simulink model "Modele_Non_Lineaire_Asservi"  (R2024a)
settings: Solver=FixedStepAuto  StartTime=0.0  StopTime=30  FixedStep=0.01  RelTol=1e-3
values from neighbouring files (symbols this model uses):
  delay = 0    [Code.m]
  den_mot_simu = [R_m*J_eq  (R_m*B_eq+n_g*n_m*k_m*k_t*K_g.^2)]    [Code.m]    (also in Initialisation.m)
  Fig_in = 1    [Code.m]
  Frequence = pi    (= 3.14159265359)    [Code.m]
  g = 9.81    [Code.m]    (also in Initialisation.m)
  K_int = real((((-1)*den_mot(1)*(Inter^2)) + ((-1)*den_mot(2)*(Inter^1))) / (num_mot(1)))    [Code.m]    (also in Initialisation.m)
  L_plaque = 0.2750/2    (= 0.1375)    [Code.m]    (also in Initialisation.m = 0.275)
  num_mot_simu = [K_g*n_m*n_g*k_t]    [Code.m]    (also in Initialisation.m)
  r_arm = 0.0254    [Code.m]    (also in Initialisation.m)
  step_size = 0.01    [Code.m]
  Test_Position = 0.06    [Code.m]    (also in Initialisation.m)
  X_den = TF_PD_Bode_Den    [Code.m]    (also in Initialisation.m)
  X_num = TF_PD_Bode_Num    [Code.m]    (also in Initialisation.m)
settings Model: Creator=Mathys  LastModifiedBy=francoisdesautels
settings RTWCC: GPUComputeCapability=3.5

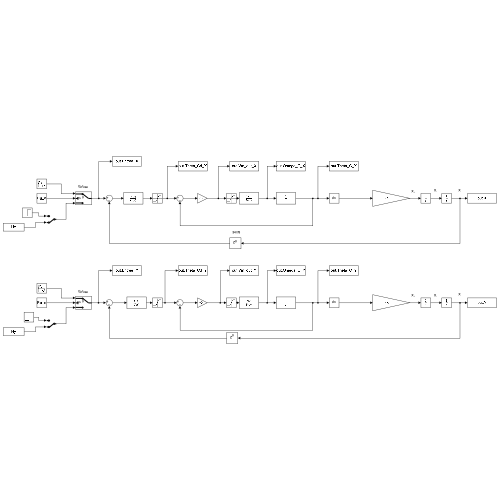
[thumbnail: Simulink's stored preview of the top-level diagram]
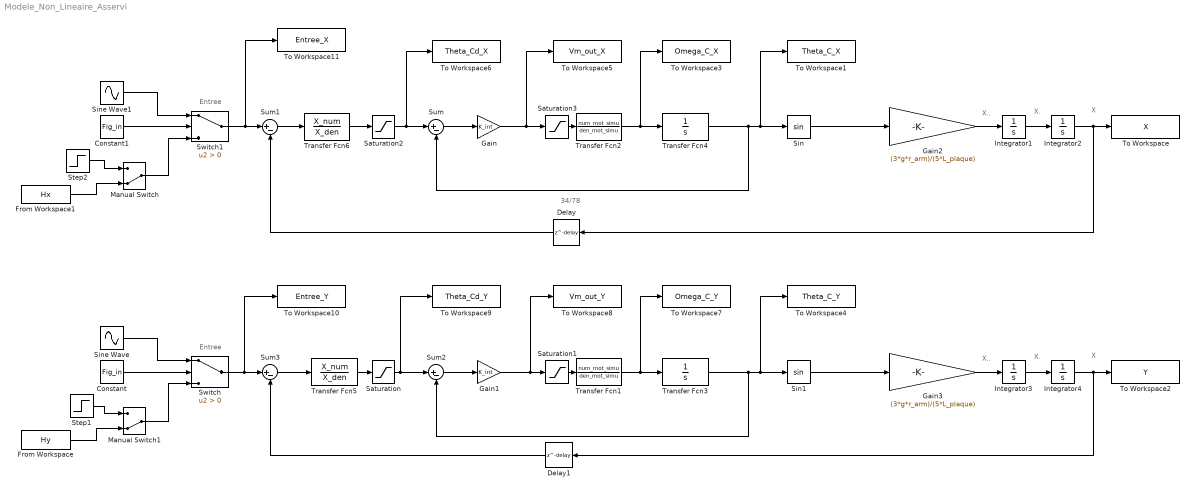
== system Modele_Non_Lineaire_Asservi ==
  note: 34/78
  note: X
  note: X.
  note: X..
  note: X..
  note: X.
  note: Entree
  note: X
  note: Entree
  Constant : Constant  Value=Fig_in
  Constant1 : Constant  Value=Fig_in
  Delay : Delay  DelayLength=delay
  Delay1 : Delay  DelayLength=delay
  From Workspace : FromWorkspace  VariableName=Hy  SampleTime=step_size
  From Workspace1 : FromWorkspace  VariableName=Hx  SampleTime=step_size
  Gain : Gain  Gain=K_int
  Gain1 : Gain  Gain=K_int
  Gain2 : Gain  Gain=(3*g*r_arm)/(5*L_plaque)
  Gain3 : Gain  Gain=(3*g*r_arm)/(5*L_plaque)
  Integrator{1..4} (4 alike) : Integrator
  Manual Switch : ManualSwitch  CurrentSetting=0
  Manual Switch1 : ManualSwitch  CurrentSetting=0
  Saturation : Saturate  UpperLimit=deg2rad(35)  LowerLimit=deg2rad(-35)
  Saturation1 : Saturate  UpperLimit=7.5  LowerLimit=-7.5
  Saturation2 : Saturate  UpperLimit=deg2rad(35)  LowerLimit=deg2rad(-35)
  Saturation3 : Saturate  UpperLimit=7.5  LowerLimit=-7.5
  Sin : Trigonometry
  Sin1 : Trigonometry
  Sine Wave : Sin  Amplitude=Test_Position  Frequency=Frequence  SampleTime=0
  Sine Wave1 : Sin  Amplitude=Test_Position  Frequency=Frequence  SampleTime=0
  Step1 : Step  After=Test_Position  SampleTime=0
  Step2 : Step  After=Test_Position  SampleTime=0
  Sum{,1..3} (4 alike) : Sum  Inputs=|+-
  Switch : Switch  Criteria=u2 > Threshold  SaturateOnIntegerOverflow=off  InputSameDT=off
  Switch1 : Switch  Criteria=u2 > Threshold  SaturateOnIntegerOverflow=off  InputSameDT=off
  To Workspace : ToWorkspace  VariableName=X  SampleTime=-1
  To Workspace1 : ToWorkspace  VariableName=Theta_C_X  SaveFormat=Timeseries  SampleTime=-1
      settings: Save2DSignal=2-D array (concatenate along first dimension)
  To Workspace10 : ToWorkspace  VariableName=Entree_Y  SaveFormat=Timeseries  SampleTime=-1
      settings: Save2DSignal=2-D array (concatenate along first dimension)
  To Workspace11 : ToWorkspace  VariableName=Entree_X  SaveFormat=Timeseries  SampleTime=-1
      settings: Save2DSignal=2-D array (concatenate along first dimension)
  To Workspace2 : ToWorkspace  VariableName=Y  SampleTime=-1
  To Workspace3 : ToWorkspace  VariableName=Omega_C_X  SampleTime=-1
  To Workspace4 : ToWorkspace  VariableName=Theta_C_Y  SaveFormat=Timeseries  SampleTime=-1
      settings: Save2DSignal=2-D array (concatenate along first dimension)
  To Workspace5 : ToWorkspace  VariableName=Vm_out_X  SaveFormat=Timeseries  SampleTime=-1
      settings: Save2DSignal=2-D array (concatenate along first dimension)
  To Workspace6 : ToWorkspace  VariableName=Theta_Cd_X  SaveFormat=Timeseries  SampleTime=-1
      settings: Save2DSignal=2-D array (concatenate along first dimension)
  To Workspace7 : ToWorkspace  VariableName=Omega_C_Y  SampleTime=-1
  To Workspace8 : ToWorkspace  VariableName=Vm_out_Y  SaveFormat=Timeseries  SampleTime=-1
      settings: Save2DSignal=2-D array (concatenate along first dimension)
  To Workspace9 : ToWorkspace  VariableName=Theta_Cd_Y  SaveFormat=Timeseries  SampleTime=-1
      settings: Save2DSignal=2-D array (concatenate along first dimension)
  Transfer Fcn1 : TransferFcn  Numerator=num_mot_simu  Denominator=den_mot_simu
  Transfer Fcn2 : TransferFcn  Numerator=num_mot_simu  Denominator=den_mot_simu
  Transfer Fcn3 : TransferFcn  Denominator=[1 0]
  Transfer Fcn4 : TransferFcn  Denominator=[1 0]
  Transfer Fcn5 : TransferFcn  Numerator=X_num  Denominator=X_den
  Transfer Fcn6 : TransferFcn  Numerator=X_num  Denominator=X_den
  wires:
  Sin/1 -> Gain2/1
  Gain2/1 -> Integrator1/1
  Integrator1/1 -> Integrator2/1
  Integrator2/1 -> Delay/1, To Workspace/1
  Transfer Fcn2/1 -> To Workspace3/1, Transfer Fcn4/1
  Sum/1 -> Gain/1
  Transfer Fcn4/1 -> To Workspace1/1, Sin/1, Sum/2
  Sum1/1 -> Transfer Fcn6/1
  Transfer Fcn6/1 -> Saturation2/1
  Gain/1 -> Saturation3/1, To Workspace5/1
  Transfer Fcn5/1 -> Saturation/1
  Transfer Fcn1/1 -> To Workspace7/1, Transfer Fcn3/1
  Transfer Fcn3/1 -> To Workspace4/1, Sin1/1, Sum2/2
  Integrator4/1 -> Delay1/1, To Workspace2/1
  Integrator3/1 -> Integrator4/1
  Gain3/1 -> Integrator3/1
  Gain1/1 -> Saturation1/1, To Workspace8/1
  Sum2/1 -> Gain1/1
  Sin1/1 -> Gain3/1
  Sum3/1 -> Transfer Fcn5/1
  Sine Wave/1 -> Switch/1
  Constant/1 -> Switch/2
  Switch/1 -> To Workspace10/1, Sum3/1
  Sine Wave1/1 -> Switch1/1
  Constant1/1 -> Switch1/2
  Manual Switch/1 -> Switch1/3
  Step2/1 -> Manual Switch/1
  Step1/1 -> Manual Switch1/1
  Manual Switch1/1 -> Switch/3
  Switch1/1 -> To Workspace11/1, Sum1/1
  From Workspace1/1 -> Manual Switch/2
  From Workspace/1 -> Manual Switch1/2
  Delay/1 -> Sum1/2
  Delay1/1 -> Sum3/2
  Saturation/1 -> To Workspace9/1, Sum2/1
  Saturation1/1 -> Transfer Fcn1/1
  Saturation2/1 -> To Workspace6/1, Sum/1
  Saturation3/1 -> Transfer Fcn2/1
